simulink model "crs_block"  (Simulink 7.4)
settings: Solver=ode45  StartTime=0.0  StopTime=10.0  RelTol=1e-3
settings Model: Creator=Mason  LastModifiedBy=Mason

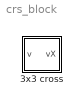
== system crs_block ==
  3x3 cross : Subsystem

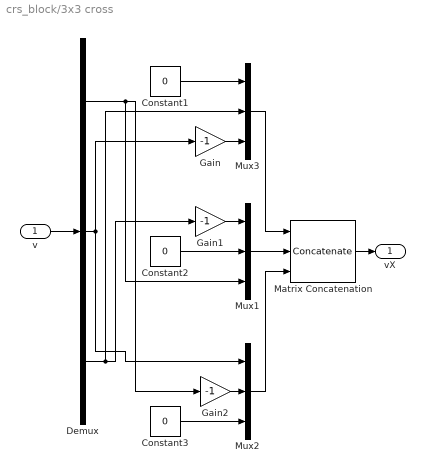
== system crs_block/3x3 cross ==
  v : Inport  OutDataType=sfix(16)  OutScaling=2^0
  Constant1 : Constant  Value=0  OutDataType=sfix(16)  OutScaling=2^0
  Constant2 : Constant  Value=0  OutDataType=sfix(16)  OutScaling=2^0
  Constant3 : Constant  Value=0  OutDataType=sfix(16)  OutScaling=2^0
  Demux : Demux  Outputs=3
  Gain : Gain  Gain=-1  ParameterDataType=sfix(16)  ParameterScaling=2^0  OutDataType=sfix(16)  OutScaling=2^0  SaturateOnIntegerOverflow=on  OutDataTypeStr=Inherit: Same as input  ParamDataTypeStr=Inherit: Same as input
  Gain1 : Gain  Gain=-1  ParameterDataType=sfix(16)  ParameterScaling=2^0  OutDataType=sfix(16)  OutScaling=2^0  SaturateOnIntegerOverflow=on  OutDataTypeStr=Inherit: Same as input  ParamDataTypeStr=Inherit: Same as input
  Gain2 : Gain  Gain=-1  ParameterDataType=sfix(16)  ParameterScaling=2^0  OutDataType=sfix(16)  OutScaling=2^0  SaturateOnIntegerOverflow=on  OutDataTypeStr=Inherit: Same as input  ParamDataTypeStr=Inherit: Same as input
  Matrix Concatenation : Concatenate  NumInputs=3  Mode=Multidimensional array  ConcatenateDimension=2
  Mux1 : Mux  Inputs=3
  Mux2 : Mux  Inputs=3
  Mux3 : Mux  Inputs=3
  vX : Outport  OutDataType=sfix(16)  OutScaling=2^0
  wires:
  v/1 -> Demux/1
  Matrix Concatenation/1 -> vX/1
  Mux3/1 -> Matrix Concatenation/1
  Mux1/1 -> Matrix Concatenation/2
  Mux2/1 -> Matrix Concatenation/3
  Gain/1 -> Mux3/3
  Gain1/1 -> Mux1/1
  Gain2/1 -> Mux2/2
  Constant1/1 -> Mux3/1
  Constant2/1 -> Mux1/2
  Constant3/1 -> Mux2/3
  Demux/3 -> Mux3/2, Gain1/1
  Demux/2 -> Gain/1, Mux2/1
  Demux/1 -> Mux1/3, Gain2/1
